simulink model "mqsls"  (R2024b)
settings: Solver=VariableStepAuto  StartTime=0.0  StopTime=10  FixedStep=0.01  RelTol=1e-3
settings Model: Creator=yangyu  LastModifiedBy=yangyu

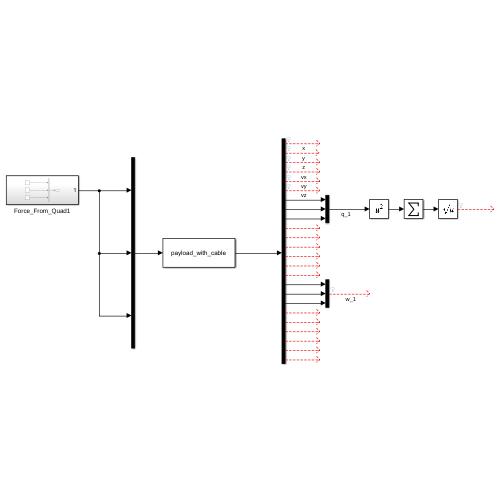
[thumbnail: Simulink's stored preview of the top-level diagram]
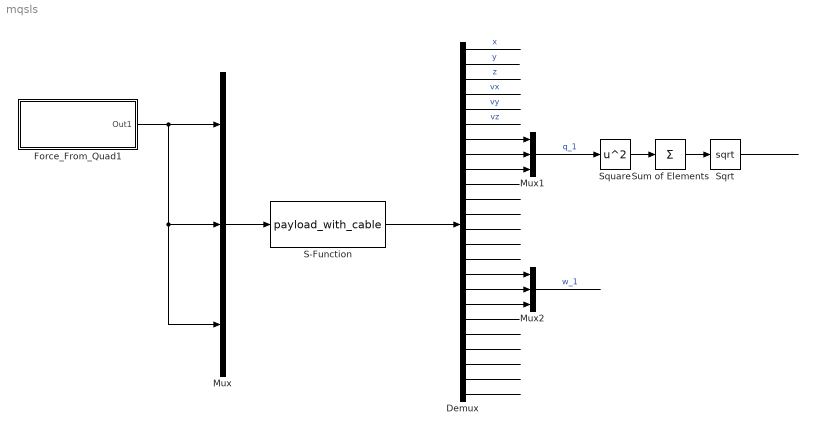
== system mqsls ==
  Demux : Demux  Outputs=24
  Force_From_Quad1 : Subsystem
  Mux : Mux  Inputs=3
  Mux1 : Mux  Inputs=3
  Mux2 : Mux  Inputs=3
  S-Function : S-Function  FunctionName=payload_with_cable  SFunctionDeploymentMode=off  EnableBusSupport=off
  Sqrt : Sqrt
  Square : Math  Operator=square
  Sum of Elements : Sum  Inputs=+
  wires:
  Mux/1 -> S-Function/1
  S-Function/1 -> Demux/1
  Demux/1 -> ?  "x"
  Demux/2 -> ?  "y"
  Demux/3 -> ?  "z"
  Force_From_Quad1/1(Out1) -> Mux/3, Mux/2, Mux/1
  Demux/4 -> ?  "vx"
  Demux/5 -> ?  "vy"
  Demux/6 -> ?  "vz"
  Demux/7 -> Mux1/1
  Demux/9 -> Mux1/3
  Demux/8 -> Mux1/2
  Demux/11 -> ?
  Demux/10 -> ?
  Demux/12 -> ?
  Demux/13 -> ?
  Demux/14 -> ?
  Demux/15 -> ?
  Demux/24 -> ?
  Demux/23 -> ?
  Demux/22 -> ?
  Demux/21 -> ?
  Demux/20 -> ?
  Demux/19 -> ?
  Mux1/1 -> Square/1  "q_1"
  Square/1 -> Sum of Elements/1
  Sum of Elements/1 -> Sqrt/1
  Sqrt/1 -> ?
  Demux/17 -> Mux2/2
  Demux/16 -> Mux2/1
  Demux/18 -> Mux2/3
  Mux2/1 -> ?  "w_1"

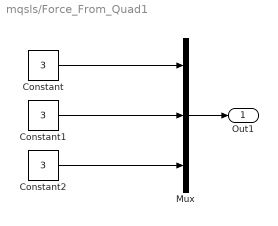
== system mqsls/Force_From_Quad1 ==
  Constant : Constant  Value=3
  Constant1 : Constant  Value=3
  Constant2 : Constant  Value=3
  Mux : Mux  Inputs=3
  Out1 : Outport
  wires:
  Mux/1 -> Out1/1
  Constant/1 -> Mux/1
  Constant1/1 -> Mux/2
  Constant2/1 -> Mux/3
